simulink model "StateSwitch_NoStateFlow"  (Simulink 8.2)
settings: Solver=FixedStepDiscrete  StartTime=0.0  StopTime=5  FixedStep=Ts  RelTol=1e-3
undefined symbols (not defined in the file): DiscIntNeverNeededParam, Ts
libraries: simulink x6
settings Model: Creator=LukePH  LastModifiedBy=LukePH
settings DataIOCC: SignalLoggingSaveFormat=Dataset
settings OptimizationCC: ExpressionDepthLimit=128
settings DebuggingCC: FcnCallInpInsideContextMsg=EnableAllAsError  StateNameClashWarn=none
settings GRTTargetCC: CombineOutputUpdateFcns=on  GRTInterface=off

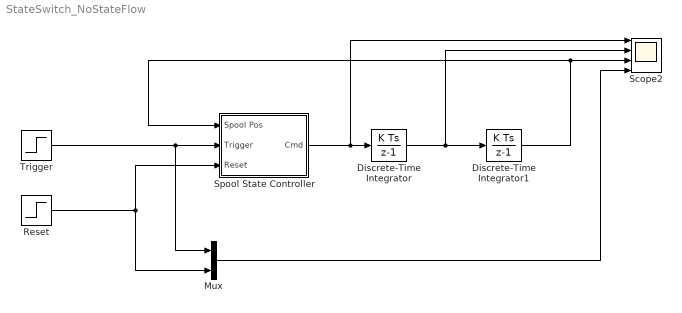
== system StateSwitch_NoStateFlow ==
  Discrete-Time Integrator : DiscreteIntegrator  SampleTime=Ts  ICPrevOutput=DiscIntNeverNeededParam  ICPrevScaledInput=DiscIntNeverNeededParam
  Discrete-Time Integrator1 : DiscreteIntegrator  SampleTime=Ts  ICPrevOutput=DiscIntNeverNeededParam  ICPrevScaledInput=DiscIntNeverNeededParam
  Mux : Mux  Inputs=2
  Reset : Step  Time=.1  Before=1  After=0  SampleTime=0
  Scope2 : Scope  NumInputPorts=4
      settings: TimeRange=5  YMin=-10~0~0~0  YMax=10~10~40~1  SaveName=ScopeData2
  Spool State Controller : Subsystem
  Trigger : Step  Time=.2  SampleTime=0
  wires:
  Spool State Controller/1(Cmd) -> Scope2/1, Discrete-Time Integrator/1
  Discrete-Time Integrator/1 -> Scope2/2, Discrete-Time Integrator1/1
  Discrete-Time Integrator1/1 -> Spool State Controller/1(Spool Pos), Scope2/3
  Trigger/1 -> Spool State Controller/2(Trigger), Mux/1
  Reset/1 -> Spool State Controller/3(Reset), Mux/2
  Mux/1 -> Scope2/4

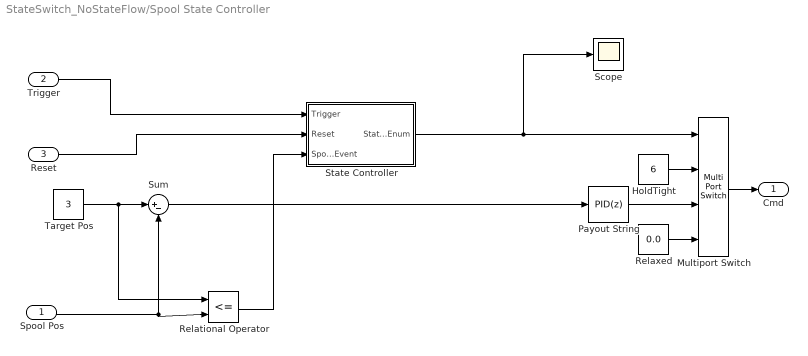
== system StateSwitch_NoStateFlow/Spool State Controller ==
  Spool Pos : Inport
  Trigger : Inport  Port=2
  Reset : Inport  Port=3
  HoldTight : Constant  Value=6
  Multiport Switch : MultiPortSwitch  DiagnosticForDefault=None
  Payout String : simulink/Continuous/PID Controller  Controller=PID  TimeDomain=Discrete-time  SampleTime=Ts  IntegratorMethod=Forward Euler  FilterMethod=Forward Euler  Form=Parallel  P=40  I=.25  D=.4  N=100  InitialConditionSource=internal  InitialConditionForIntegrator=0  InitialConditionForFilter=0  ExternalReset=none  LimitOutput=on  UpperSaturationLimit=6  LowerSaturationLimit=-6  LinearizeAsGain=off  AntiWindupMode=clamping  Kb=1  TrackingMode=off  Kt=1  PParamMin=[]  PParamMax=[]  IParamMin=[]  IParamMax=[]  DParamMin=[]  DParamMax=[]  NParamMin=[]  NParamMax=[]  KbParamMin=[]  KbParamMax=[]  KtParamMin=[]  KtParamMax=[]  POutMin=[]  POutMax=[]  IOutMin=[]  IOutMax=[]  DOutMin=[]  DOutMax=[]  NOutMin=[]  NOutMax=[]  KbOutMin=[]  KbOutMax=[]  KtOutMin=[]  KtOutMax=[]  IntegratorOutMin=[]  IntegratorOutMax=[]  FilterOutMin=[]  FilterOutMax=[]  SumOutMin=[]  SumOutMax=[]  SumI1OutMin=[]  SumI1OutMax=[]  SumI2OutMin=[]  SumI2OutMax=[]  SumI3OutMin=[]  SumI3OutMax=[]  SumDOutMin=[]  SumDOutMax=[]  SaturationOutMin=[]  SaturationOutMax=[]  IntegratorContinuousStateAttributes=''  IntegratorStateMustResolveToSignalObject=off  IntegratorRTWStateStorageClass=Auto  FilterContinuousStateAttributes=''  FilterStateMustResolveToSignalObject=off  FilterRTWStateStorageClass=Auto
  Relational Operator : RelationalOperator  Operator=<=  OutDataTypeStr=boolean
  Relaxed : Constant  Value=0.0
  Scope : Scope
  State Controller : Subsystem
  Sum : Sum  Inputs=|+-
  Target Pos : Constant  Value=3
  Cmd : Outport
  wires:
  Sum/1 -> Payout String/1
  Payout String/1 -> Multiport Switch/3
  HoldTight/1 -> Multiport Switch/2
  Relaxed/1 -> Multiport Switch/4
  Multiport Switch/1 -> Cmd/1
  Target Pos/1 -> Relational Operator/1, Sum/1
  Spool Pos/1 -> Sum/2, Relational Operator/2
  Trigger/1 -> State Controller/1(Trigger)
  Reset/1 -> State Controller/2(Reset)
  Relational Operator/1 -> State Controller/3(Spool Event)
  State Controller/1(State Enum) -> Scope/1, Multiport Switch/1

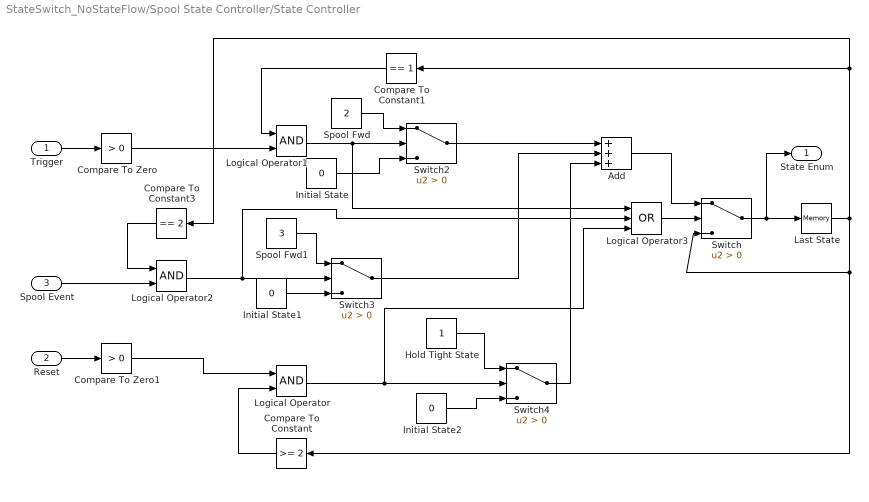
== system StateSwitch_NoStateFlow/Spool State Controller/State Controller ==
  Trigger : Inport
  Reset : Inport  Port=2
  Spool Event : Inport  Port=3
  Add : Sum  Inputs=+++
  Compare To Constant : simulink/Logic and Bit Operations/Compare To Constant  relop=>=  const=2  OutDataTypeStr=boolean
  Compare To Constant1 : simulink/Logic and Bit Operations/Compare To Constant  relop===  const=1  OutDataTypeStr=boolean
  Compare To Constant3 : simulink/Logic and Bit Operations/Compare To Constant  relop===  const=2  OutDataTypeStr=boolean
  Compare To Zero : simulink/Logic and Bit Operations/Compare To Zero  relop=>  OutDataTypeStr=boolean
  Compare To Zero1 : simulink/Logic and Bit Operations/Compare To Zero  relop=>  OutDataTypeStr=boolean
  Hold Tight State : Constant
  Initial State : Constant  Value=0
  Initial State1 : Constant  Value=0
  Initial State2 : Constant  Value=0
  Last State : Memory  X0=3
  Logical Operator : Logic  AllPortsSameDT=off  OutDataTypeStr=boolean
  Logical Operator1 : Logic  AllPortsSameDT=off  OutDataTypeStr=boolean
  Logical Operator2 : Logic  AllPortsSameDT=off  OutDataTypeStr=boolean
  Logical Operator3 : Logic  Operator=OR  Inputs=3  AllPortsSameDT=off  OutDataTypeStr=boolean
  Spool Fwd : Constant  Value=2
  Spool Fwd1 : Constant  Value=3
  Switch{,2..4} (4 alike) : Switch  Criteria=u2 > Threshold
  State Enum : Outport
  wires:
  Compare To Zero/1 -> Logical Operator1/2
  Switch/1 -> Last State/1, State Enum/1
  Trigger/1 -> Compare To Zero/1
  Reset/1 -> Compare To Zero1/1
  Compare To Constant/1 -> Logical Operator/2
  Compare To Zero1/1 -> Logical Operator/1
  Compare To Constant1/1 -> Logical Operator1/1
  Compare To Constant3/1 -> Logical Operator2/1
  Spool Event/1 -> Logical Operator2/2
  Logical Operator1/1 -> Logical Operator3/1, Switch2/2
  Spool Fwd/1 -> Switch2/1
  Logical Operator2/1 -> Logical Operator3/2, Switch3/2
  Spool Fwd1/1 -> Switch3/1
  Logical Operator/1 -> Logical Operator3/3, Switch4/2
  Hold Tight State/1 -> Switch4/1
  Logical Operator3/1 -> Switch/2
  Add/1 -> Switch/1
  Switch2/1 -> Add/1
  Switch3/1 -> Add/2
  Switch4/1 -> Add/3
  Initial State/1 -> Switch2/3
  Initial State1/1 -> Switch3/3
  Initial State2/1 -> Switch4/3
  Last State/1 -> Switch/3, Compare To Constant/1, Compare To Constant3/1, Compare To Constant1/1
